simulink model "test2"  (R2018a)
settings: Solver=VariableStepAuto  StartTime=0.0  StopTime=10.0  RelTol=1e-3
settings Model: Creator=25593  LastModifiedBy=25593

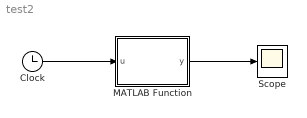
== system test2 ==
  Clock : Clock
  MATLAB Function : MATLAB Function  TreatAsAtomicUnit=on
  Scope : Scope
  wires:
  Clock/1 -> MATLAB Function/1(u)
  MATLAB Function/1(y) -> Scope/1

== matlab function test2/MATLAB Function ==
  data: u input; y output
function y = fcn(u)

y = u;
